simulink model "TEST"  (R2019a)
settings: Solver=VariableStepAuto  StartTime=0.0  StopTime=500  RelTol=1e-3
undefined symbols (not defined in the file): A, As, c, Cd, f, G, J, JD_0, Jw, Ks, L, Ls, M, m_max, q, r_ecef, t_orbit, v_ecef
libraries: vrlib x7, dspmathops x1, simulink_extras x1
(part 1 of 2)
settings Model: Creator=mario  LastModifiedBy=mario
settings DataIOCC: ReturnWorkspaceOutputs=off
settings DebuggingCC: ArithmeticOperatorsInVariantConditions=warning

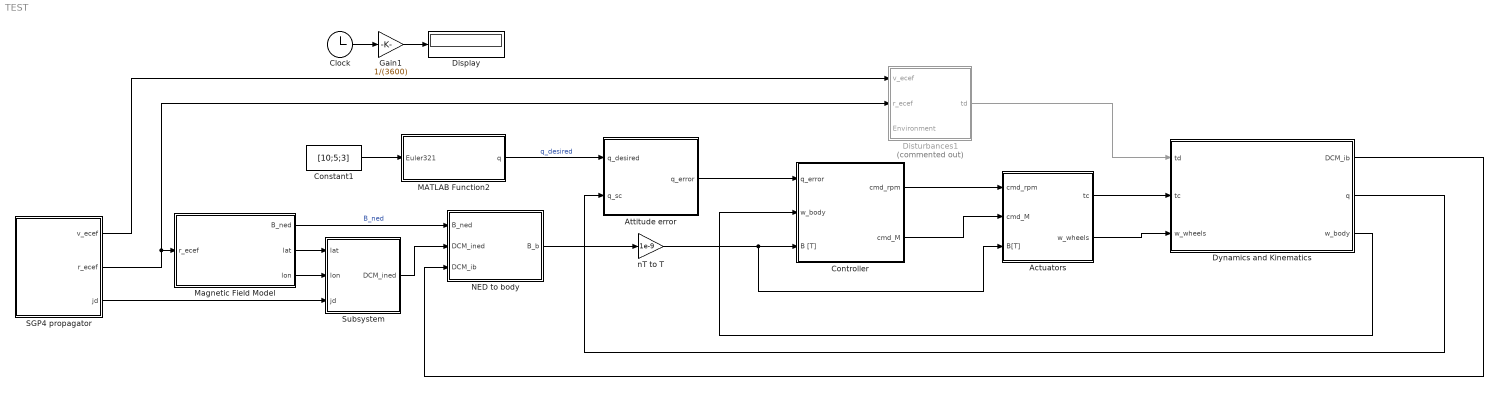
== system TEST ==
  Actuators : Subsystem
  Attitude error : Subsystem
  Clock : Clock
  Constant1 : Constant  Value=[10;5;3]
  Controller : Subsystem
  Display : Display
  Disturbances1 : Subsystem  Commented=on
  "Dynamics and Kinematics " : Subsystem
  Gain1 : Gain  Gain=1/(3600)
  MATLAB Function2 : MATLAB Function  TreatAsAtomicUnit=on
  Magnetic Field Model : Subsystem
  NED to body : Subsystem
  SGP4 propagator : Subsystem
  Subsystem : Subsystem
  nT to T : Gain  Gain=1e-9
  wires:
  "Dynamics and Kinematics "/2(q) -> Attitude error/2(q_sc)
  Constant1/1 -> MATLAB Function2/1(Euler321)
  MATLAB Function2/1(q) -> Attitude error/1(q_desired)  "q_desired"
  Controller/1("cmd_rpm ") -> Actuators/1(cmd_rpm)
  Actuators/1(tc) -> "Dynamics and Kinematics "/2(tc)
  Actuators/2(w_wheels) -> "Dynamics and Kinematics "/3(w_wheels)
  "Dynamics and Kinematics "/3(w_body) -> Controller/2(w_body)
  Attitude error/1("q_error ") -> Controller/1(q_error)
  Controller/2(cmd_M) -> Actuators/2(cmd_M)
  NED to body/1(B_b) -> nT to T/1
  nT to T/1 -> Actuators/3(B[T]), Controller/3(B [T])
  Clock/1 -> Gain1/1
  Gain1/1 -> Display/1
  Disturbances1/1(td) -> "Dynamics and Kinematics "/1(td)
  SGP4 propagator/2(r_ecef) -> Disturbances1/2("r_ecef "), Magnetic Field Model/1(r_ecef)
  "Dynamics and Kinematics "/1(DCM_ib) -> NED to body/3(DCM_ib)
  Magnetic Field Model/1(B_ned) -> NED to body/1(B_ned)  "B_ned"
  Magnetic Field Model/2(lat) -> Subsystem/1(lat)
  Magnetic Field Model/3(lon) -> Subsystem/2(lon)
  Subsystem/1(DCM_ined) -> NED to body/2(DCM_ined)
  SGP4 propagator/3(jd) -> Subsystem/3(jd)
  SGP4 propagator/1(v_ecef) -> Disturbances1/1(v_ecef)

== system TEST/Actuators ==
  cmd_rpm : Inport
  cmd_M : Inport  Port=2
  B[T] : Inport  Port=3
  Gain : Gain  Gain=0
  Magnetorquers : Subsystem
  Reaction Wheels : Subsystem
  Scope : Scope
  Sum : Sum
  tc : Outport  VectorParamsAs1DForOutWhenUnconnected=on
  w_wheels : Outport  Port=2  VectorParamsAs1DForOutWhenUnconnected=on
  wires:
  Reaction Wheels/1(t_wheels) -> Gain/1
  Reaction Wheels/2(w_wheels) -> w_wheels/1
  Magnetorquers/1(t_mtq) -> Sum/2
  Sum/1 -> Scope/1, tc/1
  cmd_rpm/1 -> Reaction Wheels/1(cmd_rpm)
  cmd_M/1 -> Magnetorquers/1(cmd_Mag)
  B[T]/1 -> Magnetorquers/2(B [T])
  Gain/1 -> Sum/1

== system TEST/Attitude error ==
  q_desired : Inport
  q_sc : Inport  Port=2
  Demux : Demux
  Gain : Gain  Gain=[1 0 0 0;0 -1 0 0;0 0 -1 0;0 0 0 -1]  Multiplication=Matrix(K*u)
  Matrix Multiply : Product  Multiplication=Matrix(*)
  Q : Subsystem
  Out Bus Element : Outport  PortName=q_error  Element=q0
  Out Bus Element1 : Outport  PortName=q_error  Element=q1
  Out Bus Element2 : Outport  PortName=q_error  Element=q2
  Out Bus Element3 : Outport  PortName=q_error  Element=q3
  wires:
  q_desired/1 -> Q/1(q)
  q_sc/1 -> Gain/1
  Q/1(Q(q)) -> Matrix Multiply/1
  Gain/1 -> Matrix Multiply/2
  Matrix Multiply/1 -> Demux/1
  Demux/1 -> Out Bus Element/1
  Demux/3 -> Out Bus Element2/1
  Demux/2 -> Out Bus Element1/1
  Demux/4 -> Out Bus Element3/1

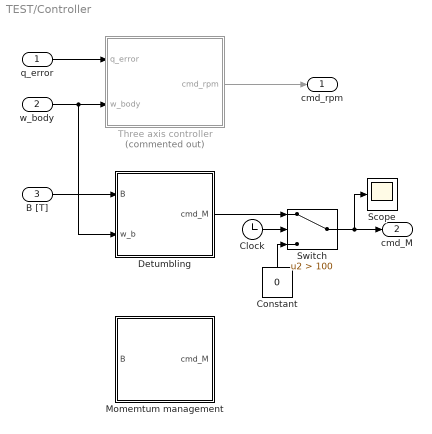
== system TEST/Controller ==
  q_error : Inport
  w_body : Inport  Port=2
  B [T] : Inport  Port=3
  Clock : Clock
  Constant : Constant  Value=0
  Detumbling : Subsystem
  Momemtum management : Subsystem
  Scope : Scope
  Switch : Switch  Criteria=u2 > Threshold  Threshold=100
  Three axis controller : Subsystem  Commented=on
  "cmd_rpm " : Outport
  cmd_M : Outport  Port=2
  wires:
  w_body/1 -> Detumbling/2(w_b), Three axis controller/2(w_body)
  q_error/1 -> Three axis controller/1(q_error)
  Three axis controller/1(cmd_rpm) -> "cmd_rpm "/1
  Detumbling/1(cmd_M) -> Switch/1
  B [T]/1 -> Detumbling/1(B)
  Switch/1 -> Scope/1, cmd_M/1
  Clock/1 -> Switch/2
  Constant/1 -> Switch/3

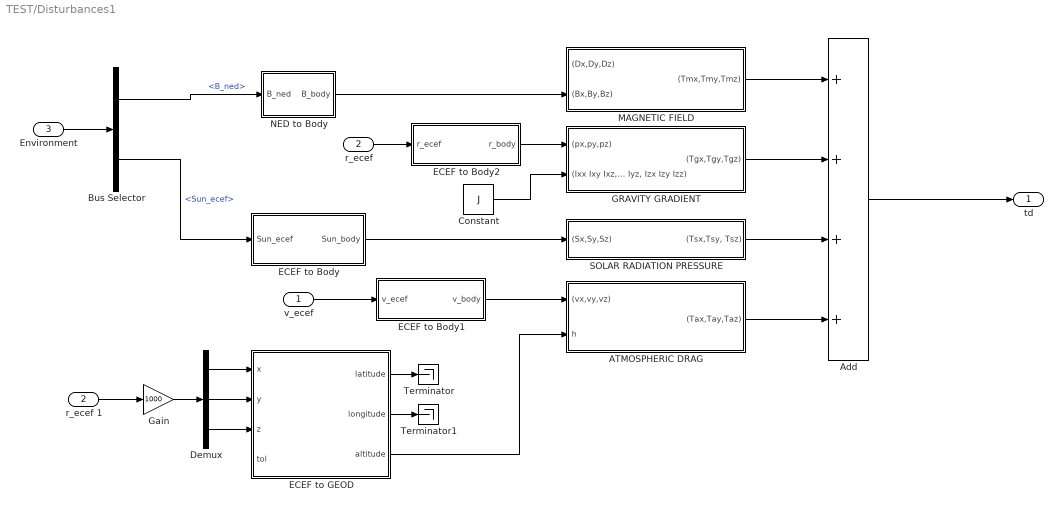
== system TEST/Disturbances1 ==
  v_ecef : Inport
  "r_ecef " : Inport  Port=2
  Environment : Inport  Port=3
  ATMOSPHERIC DRAG : Subsystem
  Add : Sum  Inputs=4
  Bus Selector : BusSelector  OutputSignals=B_ned,Sun_ecef
  Constant : Constant  Value=J
  Demux : Demux  Outputs=3
  ECEF to Body : Subsystem
  ECEF to Body1 : Subsystem
  ECEF to Body2 : Subsystem
  ECEF to GEOD : MATLAB Function  TreatAsAtomicUnit=on
  GRAVITY GRADIENT : Subsystem
  Gain : Gain  Gain=1000
  "MAGNETIC FIELD " : Subsystem
  NED to Body : Subsystem
  SOLAR RADIATION PRESSURE : Subsystem
  Terminator : Terminator
  Terminator1 : Terminator
  r_ecef 1 : InportShadow  Port=2
  td : Outport
  wires:
  Add/1 -> td/1
  ECEF to GEOD/3(altitude) -> ATMOSPHERIC DRAG/2("h ")
  Constant/1 -> GRAVITY GRADIENT/2("(Ixx Ixy Ixz, Iyx Iyy Iyz, Izx Izy Izz)")
  ATMOSPHERIC DRAG/1((Tax,Tay,Taz)) -> Add/4
  GRAVITY GRADIENT/1((Tgx,Tgy,Tgz)) -> Add/2
  ? -> "MAGNETIC FIELD "/1((Dx,Dy,Dz))
  SOLAR RADIATION PRESSURE/1("(Tsx,Tsy, Tsz)") -> Add/3
  NED to Body/1(B_body) -> "MAGNETIC FIELD "/2((Bx,By,Bz))
  "MAGNETIC FIELD "/1((Tmx,Tmy,Tmz)) -> Add/1
  ECEF to Body/1(Sun_body) -> SOLAR RADIATION PRESSURE/1((Sx,Sy,Sz))
  ECEF to Body1/1(v_body) -> ATMOSPHERIC DRAG/1((vx,vy,vz))
  Environment/1 -> Bus Selector/1
  Bus Selector/1 -> NED to Body/1(B_ned)  "<B_ned>"
  Bus Selector/2 -> ECEF to Body/1(Sun_ecef)  "<Sun_ecef>"
  v_ecef/1 -> ECEF to Body1/1(v_ecef)
  "r_ecef "/1 -> ECEF to Body2/1(r_ecef)
  ECEF to Body2/1(r_body) -> GRAVITY GRADIENT/1((px,py,pz))
  r_ecef 1/1 -> Gain/1
  Demux/1 -> ECEF to GEOD/1(x)
  Demux/2 -> ECEF to GEOD/2(y)
  Demux/3 -> ECEF to GEOD/3(z)
  ECEF to GEOD/1(latitude) -> Terminator/1
  ECEF to GEOD/2(longitude) -> Terminator1/1
  Gain/1 -> Demux/1

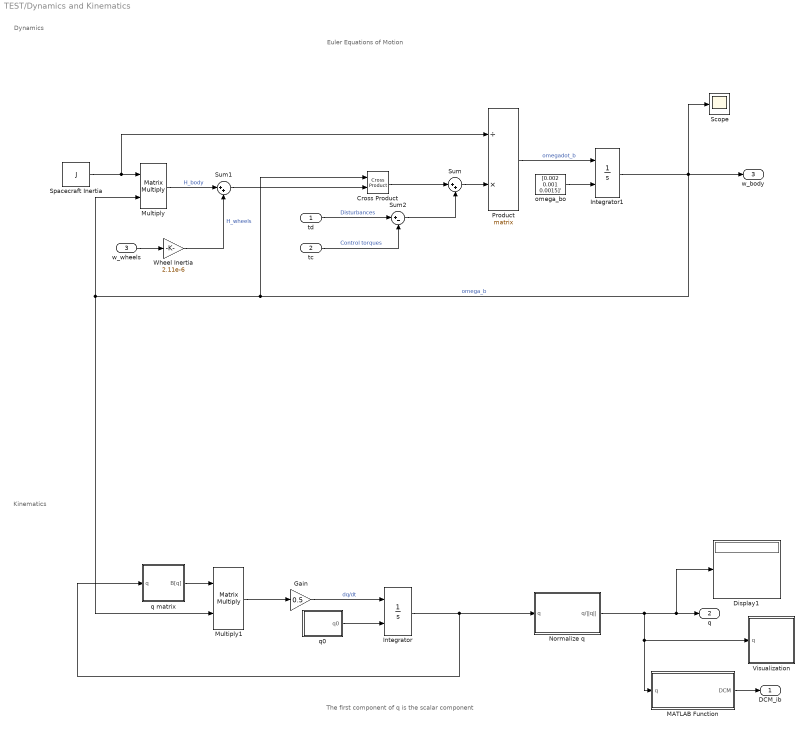
== system TEST/Dynamics and Kinematics  ==
  note: The first component of q is the scalar component
  note: Euler Equations of Motion
  note: Dynamics
  note: Kinematics
  td : Inport
  tc : Inport  Port=2
  w_wheels : Inport  Port=3
  Cross Product : vrlib/Utilities/Cross Product
      settings: SourceProductName=Simulink
  Display1 : Display
  Gain : Gain  Gain=0.5
  Integrator : Integrator  InitialConditionSource=external
  Integrator1 : Integrator  InitialConditionSource=external
  MATLAB Function : MATLAB Function  TreatAsAtomicUnit=on
  Multiply : Product  Multiplication=Matrix(*)
  Multiply1 : Product  Multiplication=Matrix(*)
  Normalize q : Subsystem
  Product : Product  Inputs=/*  Multiplication=Matrix(*)
  Scope : Scope
  Spacecraft Inertia : Constant  Value=J
  Sum : Sum  Inputs=|++
  Sum1 : Sum  Inputs=|++
  Sum2 : Sum  Inputs=|+-
  Visualization : Subsystem
  Wheel Inertia : Gain  Gain=2.11e-6
  omega_bo : Constant  Value=[0.002 0.001 0.0015]'
  q matrix : Subsystem
  q0 : Subsystem
  DCM_ib : Outport
  q : Outport  Port=2
  w_body : Outport  Port=3
  wires:
  q matrix/1(B[q]) -> Multiply1/1
  Integrator/1 -> q matrix/1(q), Normalize q/1(q)
  Gain/1 -> Integrator/1  "dq/dt"
  Multiply1/1 -> Gain/1
  Sum2/1 -> Sum/2
  Wheel Inertia/1 -> Sum1/2  "H_wheels"
  Sum1/1 -> Cross Product/2
  Cross Product/1 -> Sum/1
  Sum/1 -> Product/2
  Multiply/1 -> Sum1/1  "H_body"
  Product/1 -> Integrator1/1  "omegadot_b"
  omega_bo/1 -> Integrator1/2
  Spacecraft Inertia/1 -> Multiply/1, Product/1
  Integrator1/1 -> Scope/1, w_body/1, Multiply1/2, Multiply/2, Cross Product/1  "omega_b"
  Normalize q/1(q/||q||) -> Visualization/1(q), MATLAB Function/1(q), Display1/1, q/1
  q0/1(q0) -> Integrator/2
  td/1 -> Sum2/1  "Disturbances"
  tc/1 -> Sum2/2  "Control torques"
  w_wheels/1 -> Wheel Inertia/1
  MATLAB Function/1(DCM) -> DCM_ib/1

== system TEST/Magnetic Field Model ==
  r_ecef : Inport
  Demux : Demux  Outputs=3
  ECEF to GEOD : MATLAB Function  TreatAsAtomicUnit=on
  IGRF 13th Gen. : MATLAB Function  TreatAsAtomicUnit=on
  Mux : Mux  Inputs=3
  km to m : Gain  Gain=1000
  norm : Subsystem
  B_ned : Outport  VectorParamsAs1DForOutWhenUnconnected=on
  lat : Outport  Port=2
  lon : Outport  Port=3
  wires:
  IGRF 13th Gen./2(Be) -> Mux/2
  IGRF 13th Gen./3(Bd) -> Mux/3
  ECEF to GEOD/2(longitude) -> lon/1, IGRF 13th Gen./2(longitude)
  Demux/2 -> ECEF to GEOD/2(y)
  IGRF 13th Gen./1(Bn) -> Mux/1
  ECEF to GEOD/1(latitude) -> lat/1, IGRF 13th Gen./1(latitude)
  Demux/3 -> ECEF to GEOD/3(z)
  Demux/1 -> ECEF to GEOD/1(x)
  Mux/1 -> B_ned/1
  km to m/1 -> Demux/1
  norm/1(Out1) -> IGRF 13th Gen./3(altitude)
  r_ecef/1 -> norm/1(In1), km to m/1

== system TEST/NED to body ==
  B_ned : Inport
  DCM_ined : Inport  Port=2
  DCM_ib : Inport  Port=3
  Matrix Multiply : Product  Multiplication=Matrix(*)
  Matrix Multiply1 : Product  Multiplication=Matrix(*)
  Transpose : Math  Operator=transpose  SaturateOnIntegerOverflow=on
  B_b : Outport
  wires:
  Matrix Multiply/1 -> B_b/1
  B_ned/1 -> Matrix Multiply/2
  DCM_ib/1 -> Matrix Multiply1/1
  DCM_ined/1 -> Transpose/1
  Transpose/1 -> Matrix Multiply1/2  "DCM_nedi"
  Matrix Multiply1/1 -> Matrix Multiply/1

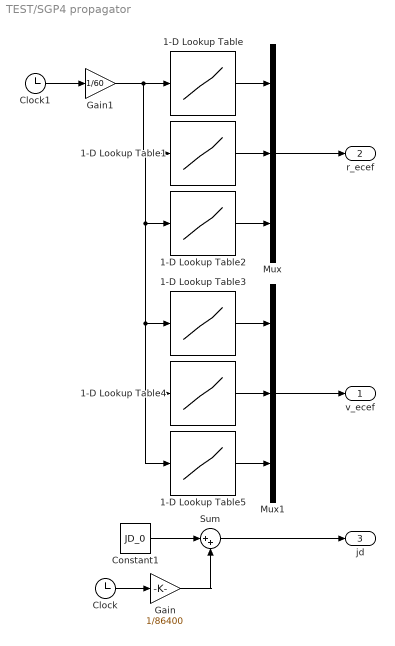
== system TEST/SGP4 propagator ==
  1-D Lookup Table : Lookup_n-D  NumberOfTableDimensions=1  BreakpointsForDimension1=t_orbit  BreakpointsForDimension2=t_orbit  BreakpointsForDimension3=t_orbit  Table=r_ecef(:,1)  InternalRulePriority=Speed  RndMeth=Simplest  InputSameDT=on
  1-D Lookup Table1 : Lookup_n-D  NumberOfTableDimensions=1  BreakpointsForDimension1=t_orbit  BreakpointsForDimension2=t_orbit  BreakpointsForDimension3=t_orbit  Table=r_ecef(:,2)  InternalRulePriority=Speed  RndMeth=Simplest  InputSameDT=on
  1-D Lookup Table2 : Lookup_n-D  NumberOfTableDimensions=1  BreakpointsForDimension1=t_orbit  BreakpointsForDimension2=t_orbit  BreakpointsForDimension3=t_orbit  Table=r_ecef(:,3)  InternalRulePriority=Speed  RndMeth=Simplest  InputSameDT=on
  1-D Lookup Table3 : Lookup_n-D  NumberOfTableDimensions=1  BreakpointsForDimension1=t_orbit  BreakpointsForDimension2=t_orbit  BreakpointsForDimension3=t_orbit  Table=v_ecef(:,1)  InternalRulePriority=Speed  RndMeth=Simplest  InputSameDT=on
  1-D Lookup Table4 : Lookup_n-D  NumberOfTableDimensions=1  BreakpointsForDimension1=t_orbit  BreakpointsForDimension2=t_orbit  BreakpointsForDimension3=t_orbit  Table=v_ecef(:,2)  InternalRulePriority=Speed  RndMeth=Simplest  InputSameDT=on
  1-D Lookup Table5 : Lookup_n-D  NumberOfTableDimensions=1  BreakpointsForDimension1=t_orbit  BreakpointsForDimension2=t_orbit  BreakpointsForDimension3=t_orbit  Table=v_ecef(:,3)  InternalRulePriority=Speed  RndMeth=Simplest  InputSameDT=on
  Clock : Clock
  Clock1 : Clock
  Constant1 : Constant  Value=JD_0
  Gain : Gain  Gain=1/86400
  Gain1 : Gain  Gain=1/60
  Mux : Mux  Inputs=3
  Mux1 : Mux  Inputs=3
  Sum : Sum  Inputs=|++
  v_ecef : Outport
  r_ecef : Outport  Port=2  VectorParamsAs1DForOutWhenUnconnected=on
  jd : Outport  Port=3
  wires:
  1-D Lookup Table2/1 -> Mux/3
  Gain1/1 -> 1-D Lookup Table5/1, 1-D Lookup Table4/1, 1-D Lookup Table3/1, 1-D Lookup Table2/1, 1-D Lookup Table1/1, 1-D Lookup Table/1
  Clock1/1 -> Gain1/1
  1-D Lookup Table1/1 -> Mux/2
  1-D Lookup Table/1 -> Mux/1
  Mux/1 -> r_ecef/1
  1-D Lookup Table3/1 -> Mux1/1
  1-D Lookup Table4/1 -> Mux1/2
  1-D Lookup Table5/1 -> Mux1/3
  Mux1/1 -> v_ecef/1
  Sum/1 -> jd/1
  Gain/1 -> Sum/2
  Constant1/1 -> Sum/1
  Clock/1 -> Gain/1

== system TEST/Subsystem ==
  lat : Inport
  lon : Inport  Port=2
  jd : Inport  Port=3
  Local Sidereal Time : MATLAB Function  TreatAsAtomicUnit=on
  MATLAB Function1 : MATLAB Function  TreatAsAtomicUnit=on
  Terminator : Terminator
  DCM_ined : Outport
  wires:
  MATLAB Function1/1(DCM_ined) -> DCM_ined/1
  Local Sidereal Time/1(lst) -> MATLAB Function1/2(lon_i)
  lat/1 -> MATLAB Function1/1(lat_d)
  lon/1 -> Local Sidereal Time/1(lon)
  jd/1 -> Local Sidereal Time/2(jd)
  Local Sidereal Time/2(gst) -> Terminator/1

== system TEST/Actuators/Magnetorquers ==
  cmd_Mag : Inport
  B [T] : Inport  Port=2
  Cross Product : vrlib/Utilities/Cross Product
      settings: SourceProductName=Simulink
  Saturation : Saturate  UpperLimit=m_max+10  LowerLimit=-m_max-10
  Scope : Scope
  Scope1 : Scope
  t_mtq : Outport
  wires:
  B [T]/1 -> Cross Product/2
  Cross Product/1 -> Scope/1, t_mtq/1
  cmd_Mag/1 -> Saturation/1
  Saturation/1 -> Scope1/1, Cross Product/1

== system TEST/Actuators/Reaction Wheels ==
  cmd_rpm : Inport
  Demux : Demux  Outputs=3
  Mux : Mux  Inputs=3
  Mux1 : Mux  Inputs=3
  Reactionwheel_x : Subsystem
  Reactionwheel_y : Subsystem
  Reactionwheel_z : Subsystem
  t_wheels : Outport
  w_wheels : Outport  Port=2
  wires:
  Reactionwheel_y/1(t_wheels) -> Mux/2
  Reactionwheel_y/2(w_wheels) -> Mux1/2
  Demux/1 -> Reactionwheel_x/1(cmd_rpm)
  Reactionwheel_x/2(w_wheels) -> Mux1/1
  Demux/2 -> Reactionwheel_y/1(cmd_rpm)
  Demux/3 -> Reactionwheel_z/1(cmd_rpm)
  Reactionwheel_z/2(w_wheels) -> Mux1/3
  Reactionwheel_x/1(t_wheels) -> Mux/1
  Reactionwheel_z/1(t_wheels) -> Mux/3
  Mux1/1 -> w_wheels/1
  Mux/1 -> t_wheels/1
  cmd_rpm/1 -> Demux/1

== system TEST/Attitude error/Q ==
  q : Inport
  Gain : Gain  Gain=[1 0 0 0;0 1 0 0;0 0 1 0;0 0 0 1]  Multiplication=Matrix(K*u)
  Gain1 : Gain  Gain=[1 0 0 0;0 -1 0 0;0 0 -1 0;0 0 0 1]  Multiplication=Matrix(K*u)
  Gain2 : Gain  Gain=[1 0 0 0;0 -1 0 0;0 0 1 0;0 0 0 -1]  Multiplication=Matrix(K*u)
  Gain4 : Gain  Gain=[1 0 0 0;0 1 0 0;0 0 -1 0;0 0 0 -1]  Multiplication=Matrix(K*u)
  Matrix Concatenate : Concatenate  NumInputs=4  Mode=Multidimensional array  ConcatenateDimension=2
  Selector1 : Selector  InputPortWidth=4  IndexOptions=Index vector (dialog)  Indices=[4 3 2 1]  OutputSizes=1
  Selector2 : Selector  InputPortWidth=4  IndexOptions=Index vector (dialog)  Indices=[2 1 4 3]  OutputSizes=1
  Selector4 : Selector  InputPortWidth=4  IndexOptions=Index vector (dialog)  Indices=[3 4 1 2]  OutputSizes=1
  Q(q) : Outport
  wires:
  Gain1/1 -> Selector2/1
  Gain/1 -> Matrix Concatenate/1
  q/1 -> Gain2/1, Gain4/1, Gain1/1, Gain/1
  Selector4/1 -> Matrix Concatenate/3
  Matrix Concatenate/1 -> Q(q)/1
  Selector2/1 -> Matrix Concatenate/2
  Gain4/1 -> Selector4/1
  Gain2/1 -> Selector1/1
  Selector1/1 -> Matrix Concatenate/4

== system TEST/Controller/Detumbling ==
  B : Inport
  w_b : Inport  Port=2
  Bang-Bang : Subsystem
  Cross Product : vrlib/Utilities/Cross Product
      settings: SourceProductName=Simulink
  Divide : Product  Inputs=*/
  Gain : Gain  Gain=-1
  Scope : Scope
  Scope1 : Scope
  norm : Subsystem
  cmd_M : Outport
  wires:
  Bang-Bang/1(Out1) -> Scope/1
  B/1 -> Cross Product/2, norm/1(B), Bang-Bang/1(In1)
  w_b/1 -> Cross Product/1
  norm/1(||B||) -> Divide/2
  Cross Product/1 -> Divide/1
  Divide/1 -> Gain/1
  Gain/1 -> cmd_M/1, Scope1/1

== system TEST/Controller/Momemtum management ==
  B : Inport
  Sign : Signum
  cmd_M : Outport

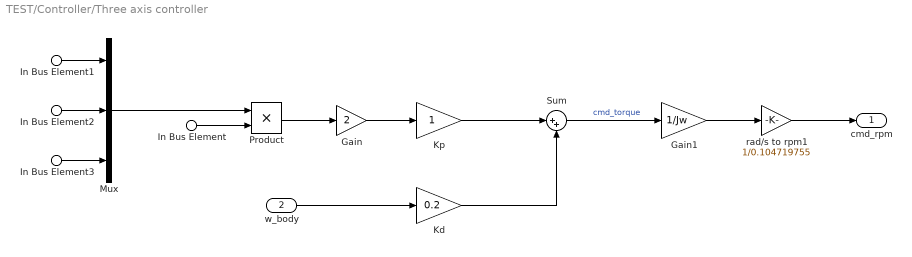
== system TEST/Controller/Three axis controller ==
  In Bus Element : Inport  PortName=q_error  Element=q0
  In Bus Element1 : Inport  PortName=q_error  Element=q1
  In Bus Element2 : Inport  PortName=q_error  Element=q2
  In Bus Element3 : Inport  PortName=q_error  Element=q3
  w_body : Inport  Port=2
  Gain : Gain  Gain=2
  Gain1 : Gain  Gain=1/Jw
  Kd : Gain  Gain=0.2
  Kp : Gain
  Mux : Mux  Inputs=3
  Product : Product
  Sum : Sum  Inputs=|++
  rad/s to rpm1 : Gain  Gain=1/0.104719755
  cmd_rpm : Outport
  wires:
  Kp/1 -> Sum/1
  w_body/1 -> Kd/1
  Product/1 -> Gain/1
  Sum/1 -> Gain1/1  "cmd_torque"
  Kd/1 -> Sum/2
  Gain1/1 -> rad/s to rpm1/1
  rad/s to rpm1/1 -> cmd_rpm/1
  Gain/1 -> Kp/1
  Mux/1 -> Product/1
  In Bus Element3/1 -> Mux/3
  In Bus Element/1 -> Product/2
  In Bus Element1/1 -> Mux/1
  In Bus Element2/1 -> Mux/2

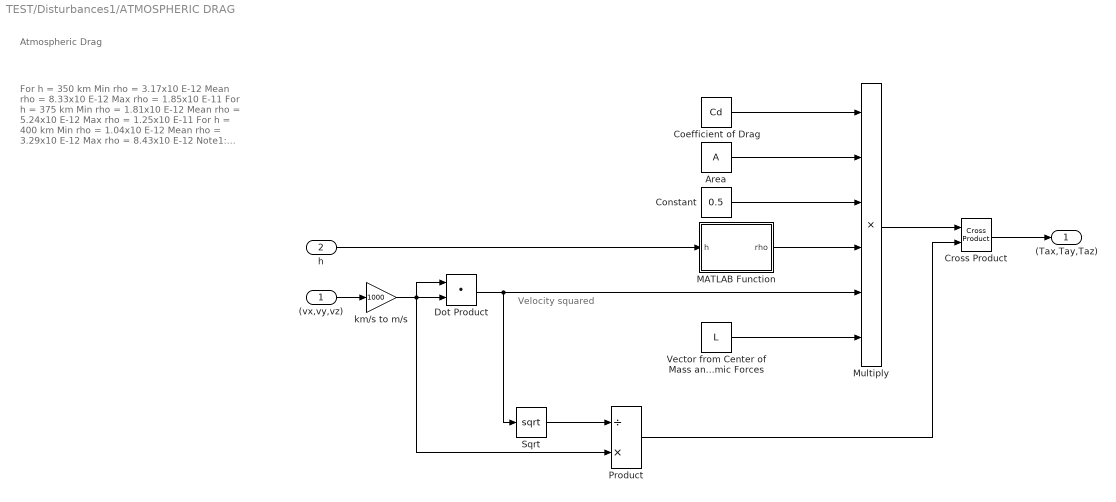
== system TEST/Disturbances1/ATMOSPHERIC DRAG ==
  note: Velocity squared
  note: For h = 350 km
      |
      | Min rho = 3.17x10 E-12
      | Mean rho = 8.33x10 E-12
      | Max rho = 1.85x10 E-11
      |
      | For h = 375 km
      |
      | Min rho = 1.81x10 E-12
      | Mean rho = 5.24x10 E-12
      | Max rho = 1.25x10 E-11
      |
      | For h = 400 km
      |
      | Min rho = 1.04x10 E-12
      | Mean rho = 3.29x10 E-12
      | Max rho = 8.43x10 E-12
      |
      | Note1: Mean Rho has an accuracy of 10%
      | Note2: Rho (kg/m^3)
      | Note3 : Rho depends on solar pressure and the solar cycle
      | Source : New SMAD p.1031
  note: Atmospheric Drag
  (vx,vy,vz) : Inport
  "h " : Inport  Port=2
  Area : Constant  Value=A
  Coefficient of Drag : Constant  Value=Cd
  Constant : Constant  Value=0.5
  Cross Product : vrlib/Utilities/Cross Product
      settings: SourceProductBaseCode=VR
  Dot Product : DotProduct  InputSameDT=on  OutDataTypeStr=Inherit: Inherit via internal rule
  MATLAB Function : MATLAB Function  TreatAsAtomicUnit=on
  Multiply : Product  Inputs=6
  Product : Product  Inputs=/*
  Sqrt : Sqrt  SaturateOnIntegerOverflow=on
  "Vector from Center of Mass and Center of Aerodynamic Forces " : Constant  Value=L
  km/s to m/s : Gain  Gain=1000
  (Tax,Tay,Taz) : Outport
  wires:
  Constant/1 -> Multiply/3
  Multiply/1 -> Cross Product/1
  (vx,vy,vz)/1 -> km/s to m/s/1
  "h "/1 -> MATLAB Function/1(h)
  Sqrt/1 -> Product/1
  Product/1 -> Cross Product/2
  Dot Product/1 -> Sqrt/1, Multiply/5
  Area/1 -> Multiply/2
  Coefficient of Drag/1 -> Multiply/1
  MATLAB Function/1(rho) -> Multiply/4
  "Vector from Center of Mass and Center of Aerodynamic Forces "/1 -> Multiply/6
  Cross Product/1 -> (Tax,Tay,Taz)/1
  km/s to m/s/1 -> Dot Product/1, Product/2, Dot Product/2

== system TEST/Disturbances1/ECEF to Body ==
  Sun_ecef : Inport
  Sun_body : Outport
  wires:
  Sun_ecef/1 -> Sun_body/1

== system TEST/Disturbances1/ECEF to Body1 ==
  v_ecef : Inport
  v_body : Outport
  wires:
  v_ecef/1 -> v_body/1

== system TEST/Disturbances1/ECEF to Body2 ==
  r_ecef : Inport
  r_body : Outport
  wires:
  r_ecef/1 -> r_body/1

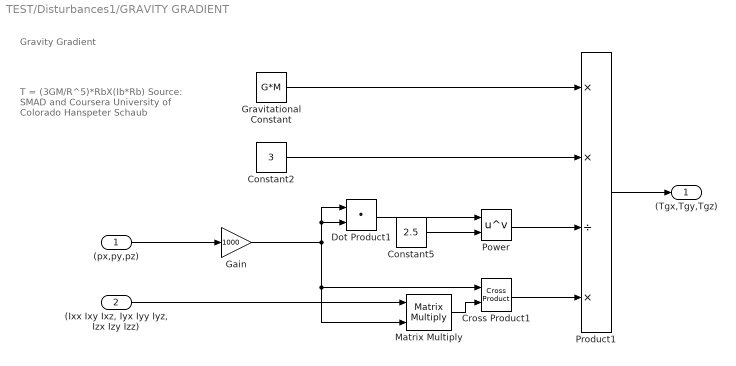
== system TEST/Disturbances1/GRAVITY GRADIENT ==
  note: T = (3GM/R^5)*RbX(Ib*Rb)
      |
      | Source: SMAD and Coursera
      | University of Colorado Hanspeter
      | Schaub
  note: Gravity Gradient
  (px,py,pz) : Inport
  "(Ixx Ixy Ixz, Iyx Iyy Iyz, Izx Izy Izz)" : Inport  Port=2
  Constant2 : Constant  Value=3
  Constant5 : Constant  Value=2.5
  Cross Product1 : vrlib/Utilities/Cross Product
      settings: SourceProductBaseCode=VR
  Dot Product1 : DotProduct  InputSameDT=on  OutDataTypeStr=Inherit: Inherit via internal rule
  Gain : Gain  Gain=1000
  Gravitational Constant : Constant  Value=G*M
  Matrix Multiply : Product  Multiplication=Matrix(*)
  Power : Math  Operator=pow  SaturateOnIntegerOverflow=on
  Product1 : Product  Inputs=**/*
  (Tgx,Tgy,Tgz) : Outport
  wires:
  (px,py,pz)/1 -> Gain/1
  Dot Product1/1 -> Power/1
  Constant5/1 -> Power/2
  Cross Product1/1 -> Product1/4
  Constant2/1 -> Product1/2
  "(Ixx Ixy Ixz, Iyx Iyy Iyz, Izx Izy Izz)"/1 -> Matrix Multiply/1
  Matrix Multiply/1 -> Cross Product1/2
  Gravitational Constant/1 -> Product1/1
  Power/1 -> Product1/3
  Product1/1 -> (Tgx,Tgy,Tgz)/1
  Gain/1 -> Matrix Multiply/2, Cross Product1/1, Dot Product1/1, Dot Product1/2

== system TEST/Disturbances1/MAGNETIC FIELD  ==
  note: Magnetic Field
  (Dx,Dy,Dz) : Inport
  (Bx,By,Bz) : Inport  Port=2
  Cross Product : vrlib/Utilities/Cross Product
      settings: SourceProductBaseCode=VR
  nT to T : Gain  Gain=1e-9
  (Tmx,Tmy,Tmz) : Outport
  wires:
  Cross Product/1 -> (Tmx,Tmy,Tmz)/1
  (Bx,By,Bz)/1 -> nT to T/1
  (Dx,Dy,Dz)/1 -> Cross Product/1
  nT to T/1 -> Cross Product/2

== system TEST/Disturbances1/NED to Body ==
  B_ned : Inport
  B_body : Outport
  wires:
  B_ned/1 -> B_body/1

== system TEST/Disturbances1/SOLAR RADIATION PRESSURE ==
  note: Solar Radiation
      | Pressure
  (Sx,Sy,Sz) : Inport
  Cross Product2 : vrlib/Utilities/Cross Product
      settings: SourceProductBaseCode=VR
  Inverse because the Force is in the opposite direction : Gain  Gain=-1
  Normalization : dspmathops/Normalization  NormType=2-norm  Bias=1e-10  NormOver=Each column  Dimension=1  roundingMode=Floor  overflowMode=off  accumDataTypeStr=Inherit: Same as product output  accumLastDataTypeStr=Inherit: Same as product output  outputDataTypeStr=Inherit: Same as product output  outputMin=[]  outputMax=[]  outputLastDataTypeStr=Inherit: Same as product output
      settings: SourceProductName=DSP System Toolbox
  Product3 : Product  Inputs=5
  Solar Constant : Constant  Value=Ks
  Speed of Light : Constant  Value=1/c
  Sunlit Area : Constant  Value=As
  Unitless Reflectance Factor : Constant  Value=1+q
  Vector from Center of Mass to Center of Solar Pressure : Constant  Value=Ls
  "(Tsx,Tsy, Tsz)" : Outport
  wires:
  Cross Product2/1 -> "(Tsx,Tsy, Tsz)"/1
  Sunlit Area/1 -> Product3/1
  Vector from Center of Mass to Center of Solar Pressure/1 -> Cross Product2/1
  (Sx,Sy,Sz)/1 -> Normalization/1
  Solar Constant/1 -> Product3/4
  Product3/1 -> Cross Product2/2
  Inverse because the Force is in the opposite direction/1 -> Product3/5
  Speed of Light/1 -> Product3/3
  Unitless Reflectance Factor/1 -> Product3/2
  Normalization/1 -> Inverse because the Force is in the opposite direction/1

== system TEST/Dynamics and Kinematics /Normalize q ==
  q : Inport
  Divide : Product  Inputs=*/
  Dot Product : DotProduct  InputSameDT=on  OutDataTypeStr=Inherit: Inherit via internal rule
  Sqrt : Sqrt  SaturateOnIntegerOverflow=on
  q/||q|| : Outport
  wires:
  Divide/1 -> q/||q||/1
  Dot Product/1 -> Sqrt/1
  Sqrt/1 -> Divide/2
  q/1 -> Dot Product/1, Dot Product/2, Divide/1

== system TEST/Dynamics and Kinematics /Visualization ==
  q : Inport
  MATLAB Function : MATLAB Function  TreatAsAtomicUnit=on
  Radians to Degrees : simulink_extras/Transformations/Radians to Degrees
  Scope : Scope
  To Workspace : ToWorkspace  VariableName=euler  SampleTime=0.05
  wires:
  Radians to Degrees/1 -> Scope/1
  MATLAB Function/1(Euler321) -> Radians to Degrees/1, To Workspace/1
  q/1 -> MATLAB Function/1(q)

== system TEST/Dynamics and Kinematics /q matrix ==
  q : Inport
  Gain : Gain  Gain=[1 0 0 0;0 -1 0 0;0 0 -1 0;0 0 0 1]  Multiplication=Matrix(K*u)
  Gain1 : Gain  Gain=[1 0 0 0;0 1 0 0;0 0 -1 0;0 0 0 -1]  Multiplication=Matrix(K*u)
  Gain4 : Gain  Gain=[1 0 0 0;0 -1 0 0;0 0 1 0;0 0 0 -1]  Multiplication=Matrix(K*u)
  Matrix Concatenate : Concatenate  NumInputs=3  Mode=Multidimensional array  ConcatenateDimension=2
  Selector : Selector  InputPortWidth=4  IndexOptions=Index vector (dialog)  Indices=[2 1 4 3]  OutputSizes=1
  Selector2 : Selector  InputPortWidth=4  IndexOptions=Index vector (dialog)  Indices=[3 4 1 2]  OutputSizes=1
  Selector4 : Selector  InputPortWidth=4  IndexOptions=Index vector (dialog)  Indices=[4 3 2 1]  OutputSizes=1
  B[q] : Outport
  wires:
  Gain/1 -> Selector/1
  Gain1/1 -> Selector2/1
  Selector/1 -> Matrix Concatenate/1
  q/1 -> Gain1/1, Gain/1, Gain4/1
  Selector4/1 -> Matrix Concatenate/3
  Matrix Concatenate/1 -> B[q]/1
  Selector2/1 -> Matrix Concatenate/2
  Gain4/1 -> Selector4/1

== system TEST/Dynamics and Kinematics /q0 ==
  Constant : Constant  Value=[0;0;0]
  MATLAB Function1 : MATLAB Function  TreatAsAtomicUnit=on
  q0 : Outport
  wires:
  Constant/1 -> MATLAB Function1/1(Euler321)
  MATLAB Function1/1(q) -> q0/1

== system TEST/Magnetic Field Model/norm ==
  In1 : Inport
  Add : Sum  Inputs=+++
  Demux : Demux  Outputs=3
  Product : Product
  Product1 : Product
  Product2 : Product
  Sqrt : Sqrt  SaturateOnIntegerOverflow=on
  Out1 : Outport
  wires:
  Demux/2 -> Product1/2, Product1/1
  Demux/1 -> Product/2, Product/1
  Sqrt/1 -> Out1/1
  Product2/1 -> Add/3
  Product1/1 -> Add/2
  Product/1 -> Add/1
  Add/1 -> Sqrt/1
  Demux/3 -> Product2/2, Product2/1
  In1/1 -> Demux/1

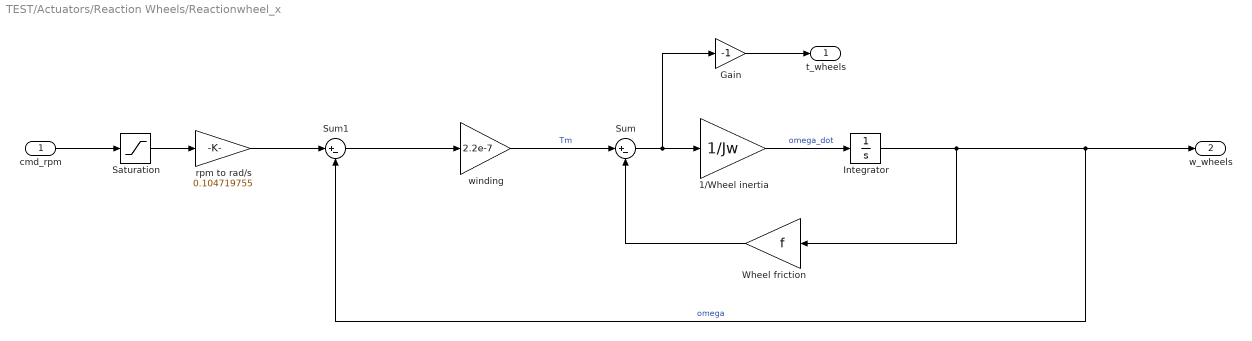
== system TEST/Actuators/Reaction Wheels/Reactionwheel_x ==
  cmd_rpm : Inport
  1/Wheel inertia : Gain  Gain=1/Jw
  Gain : Gain  Gain=-1
  Integrator : Integrator
  Saturation : Saturate  UpperLimit=8000  LowerLimit=-8000
  Sum : Sum  Inputs=|+-
  Sum1 : Sum  Inputs=|+-
  Wheel friction : Gain  Gain=f
  rpm to rad/s : Gain  Gain=0.104719755
  winding : Gain  Gain=2.2e-7
  t_wheels : Outport
  w_wheels : Outport  Port=2
  wires:
  cmd_rpm/1 -> Saturation/1
  Integrator/1 -> w_wheels/1, Sum1/2, Wheel friction/1  "omega"
  Wheel friction/1 -> Sum/2
  Sum1/1 -> winding/1
  1/Wheel inertia/1 -> Integrator/1  "omega_dot"
  winding/1 -> Sum/1  "Tm"
  Sum/1 -> Gain/1, 1/Wheel inertia/1
  rpm to rad/s/1 -> Sum1/1
  Saturation/1 -> rpm to rad/s/1
  Gain/1 -> t_wheels/1

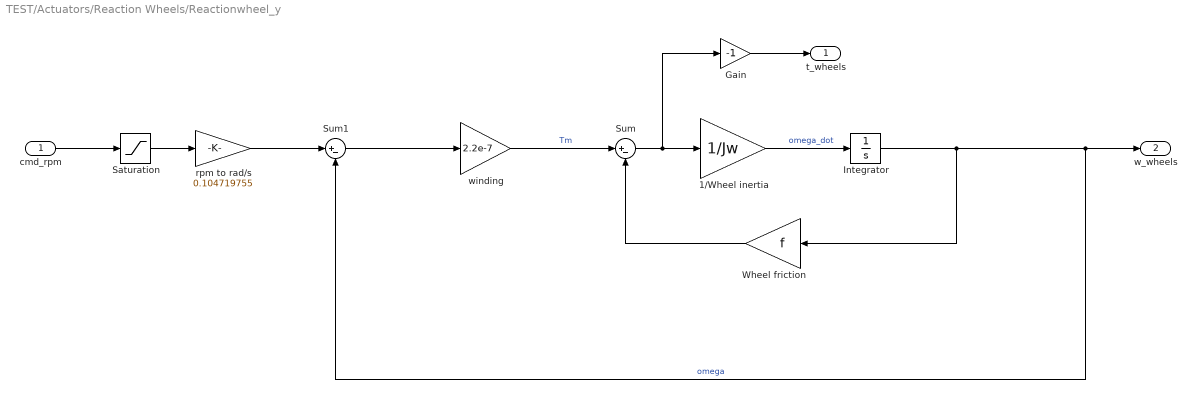
== system TEST/Actuators/Reaction Wheels/Reactionwheel_y ==
  cmd_rpm : Inport
  1/Wheel inertia : Gain  Gain=1/Jw
  Gain : Gain  Gain=-1
  Integrator : Integrator
  Saturation : Saturate  UpperLimit=8000  LowerLimit=-8000
  Sum : Sum  Inputs=|+-
  Sum1 : Sum  Inputs=|+-
  Wheel friction : Gain  Gain=f
  rpm to rad/s : Gain  Gain=0.104719755
  winding : Gain  Gain=2.2e-7
  t_wheels : Outport
  w_wheels : Outport  Port=2
  wires:
  Saturation/1 -> rpm to rad/s/1
  rpm to rad/s/1 -> Sum1/1
  Sum/1 -> 1/Wheel inertia/1, Gain/1
  winding/1 -> Sum/1  "Tm"
  1/Wheel inertia/1 -> Integrator/1  "omega_dot"
  Sum1/1 -> winding/1
  Wheel friction/1 -> Sum/2
  Integrator/1 -> Wheel friction/1, w_wheels/1, Sum1/2  "omega"
  cmd_rpm/1 -> Saturation/1
  Gain/1 -> t_wheels/1

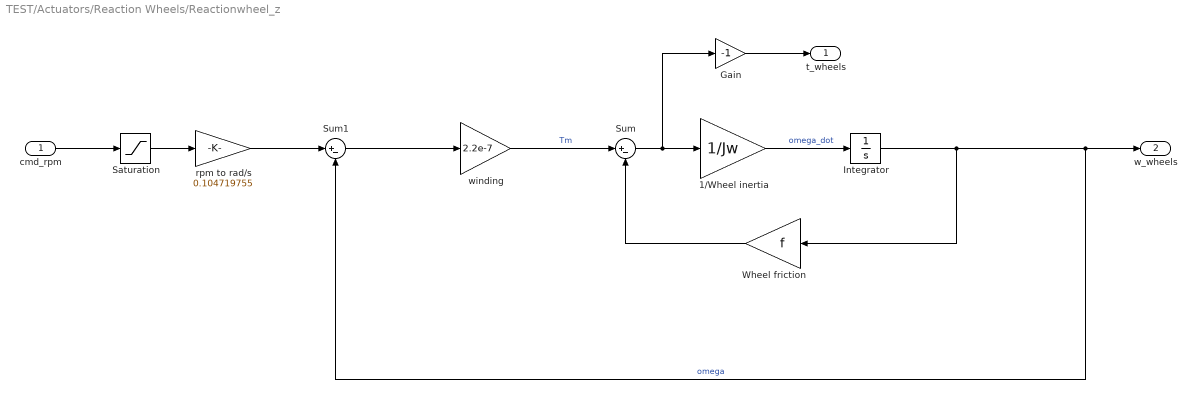
== system TEST/Actuators/Reaction Wheels/Reactionwheel_z ==
  cmd_rpm : Inport
  1/Wheel inertia : Gain  Gain=1/Jw
  Gain : Gain  Gain=-1
  Integrator : Integrator
  Saturation : Saturate  UpperLimit=8000  LowerLimit=-8000
  Sum : Sum  Inputs=|+-
  Sum1 : Sum  Inputs=|+-
  Wheel friction : Gain  Gain=f
  rpm to rad/s : Gain  Gain=0.104719755
  winding : Gain  Gain=2.2e-7
  t_wheels : Outport
  w_wheels : Outport  Port=2
  wires:
  cmd_rpm/1 -> Saturation/1
  Integrator/1 -> Sum1/2, w_wheels/1, Wheel friction/1  "omega"
  Wheel friction/1 -> Sum/2
  Sum1/1 -> winding/1
  1/Wheel inertia/1 -> Integrator/1  "omega_dot"
  winding/1 -> Sum/1  "Tm"
  Sum/1 -> Gain/1, 1/Wheel inertia/1
  rpm to rad/s/1 -> Sum1/1
  Saturation/1 -> rpm to rad/s/1
  Gain/1 -> t_wheels/1

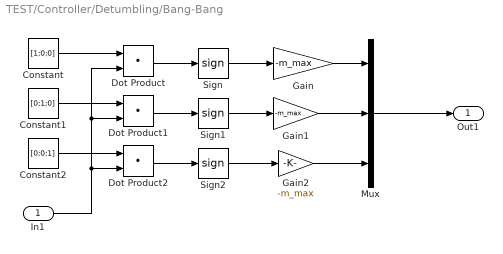
== system TEST/Controller/Detumbling/Bang-Bang ==
  In1 : Inport
  Constant : Constant  Value=[1;0;0]
  Constant1 : Constant  Value=[0;1;0]
  Constant2 : Constant  Value=[0;0;1]
  Dot Product : DotProduct  InputSameDT=on  OutDataTypeStr=Inherit: Inherit via internal rule
  Dot Product1 : DotProduct  InputSameDT=on  OutDataTypeStr=Inherit: Inherit via internal rule
  Dot Product2 : DotProduct  InputSameDT=on  OutDataTypeStr=Inherit: Inherit via internal rule
  Gain : Gain  Gain=-m_max
  Gain1 : Gain  Gain=-m_max
  Gain2 : Gain  Gain=-m_max
  Mux : Mux  Inputs=3
  Sign : Signum
  Sign1 : Signum
  Sign2 : Signum
  Out1 : Outport
  wires:
  In1/1 -> Dot Product2/2, Dot Product1/2, Dot Product/2
  Dot Product2/1 -> Sign2/1
  Sign2/1 -> Gain2/1
  Gain/1 -> Mux/1
  Sign/1 -> Gain/1
  Sign1/1 -> Gain1/1
  Constant/1 -> Dot Product/1
  Constant1/1 -> Dot Product1/1
  Dot Product/1 -> Sign/1
  Gain2/1 -> Mux/3
  Constant2/1 -> Dot Product2/1
  Dot Product1/1 -> Sign1/1
  Gain1/1 -> Mux/2
  Mux/1 -> Out1/1

== system TEST/Controller/Detumbling/norm ==
  B : Inport
  Add : Sum  Inputs=3
  Demux : Demux  Outputs=3
  Product : Product
  Product1 : Product
  Product2 : Product
  ||B|| : Outport
  wires:
  Add/1 -> ||B||/1
  Product2/1 -> Add/3
  Product1/1 -> Add/2
  Product/1 -> Add/1
  Demux/3 -> Product2/1, Product2/2
  Demux/2 -> Product1/1, Product1/2
  Demux/1 -> Product/1, Product/2
  B/1 -> Demux/1

== matlab function TEST/Dynamics and Kinematics /q0/MATLAB Function1 ==
  data: Euler321 input; q output
function q = euler3212q(Euler321)
euler = [deg2rad(Euler321(1));deg2rad(Euler321(2));deg2rad(Euler321(3))];

c1 = cos(euler(1)/2);
s1 = sin(euler(1)/2);
c2 = cos(euler(2)/2);
s2 = sin(euler(2)/2);
c3 = cos(euler(3)/2);
s3 = sin(euler(3)/2);

q = [c1*c2*c3+s1*s2*s3 ;
     s1*c2*c3-c1*s2*s3;
     c1*s2*c3+s1*c2*s3;
     c1*c2*s3-s1*s2*c3];

== matlab function TEST/Dynamics and Kinematics /Visualization/MATLAB Function ==
  data: q input; Euler321 output
function Euler321 = q2euler(q)
q1 = q(1);
qbar = [q(2);q(3);q(4)];
qtilde = [0 -qbar(3) qbar(2);qbar(3) 0 -qbar(1);-qbar(2) qbar(1) 0];

DCM = 2*(qbar*qbar') + (q1^2-qbar'*qbar)*eye(3) - 2*q1*qtilde;

Euler321 = [atan2(DCM(1,2),DCM(1,1));-asin(DCM(1,3)); atan2(DCM(2,3),DCM(3,3))];

== matlab function TEST/MATLAB Function2 ==
  data: Euler321 input; q output
function q = euler3212q(Euler321)
euler = [deg2rad(Euler321(1));deg2rad(Euler321(2));deg2rad(Euler321(3))];

c1 = cos(euler(1)/2);
s1 = sin(euler(1)/2);
c2 = cos(euler(2)/2);
s2 = sin(euler(2)/2);
c3 = cos(euler(3)/2);
s3 = sin(euler(3)/2);

q = [c1*c2*c3+s1*s2*s3 ;
     s1*c2*c3-c1*s2*s3;
     c1*s2*c3+s1*c2*s3;
     c1*c2*s3-s1*s2*c3];

== matlab function TEST/Subsystem/Local Sidereal Time ==
  data: lon input; lst output; jd input; gst output
% -----------------------------------------------------------------------------
%
%                           function lstime
%
%  this function finds the local sidereal time at a given location.
%
%  author        : david vallado                  719-573-2600   27 may 2002
%
%  revisions
%                -
%
%  inputs          description                    range / units
%    lon         - site longitude (west -)        -2pi to 2pi rad
%    jd          - julian date                    days from 4713 bc
%
%  outputs       :
%    lst         - local sidereal time            0.0 to 2pi rad
%    gst         - greenwich sidereal time        0.0 to 2pi rad
%
%  locals        :
%    none.
%
%  coupling      :
%    gstime        finds the greenwich sidereal time
%
%  references    :
%    vallado       2007, 194, alg 15, ex 3-5
%
% [lst,gst] = lstime ( lon, jd );
% -----------------------------------------------------------------------------

function [lst,gst] = lstime ( lon, jd )

        twopi  = 2.0*pi;

        % ------------------------  implementation   ------------------
        [gst] = gstime( jd );
        lst = lon + gst;

        % ----------------------- check quadrants ---------------------
        lst = rem( lst,twopi );
        if ( lst < 0.0 )
            lst= lst + twopi;
        end
          
% -----------------------------------------------------------------------------
%
%                           function gstime
%
%  this function finds the greenwich sidereal time (iau-82).
%
%  author        : david vallado                  719-573-2600    7 jun 2002
%
%  revisions
%                -
%
%  inputs          description                    range / units
%    jdut1       - julian date of ut1             days from 4713 bc
%
%  outputs       :
%    gst         - greenwich sidereal time        0 to 2pi rad
%
%  locals        :
%    temp        - temporary variable for reals   rad
%    tut1        - julian centuries from the
%                  jan 1, 2000 12 h epoch (ut1)
%
%  coupling      :
%
%  references    :
%    vallado       2007, 193, Eq 3-43
%
% gst = gstime(jdut1);
% -----------------------------------------------------------------------------

function gst = gstime(jdut1);

        twopi      = 2.0*pi;
        deg2rad    = pi/180.0;

        % ------------------------  implementation   ------------------
        tut1= ( jdut1 - 2451545.0 ) / 36525.0;

        temp = - 6.2e-6 * tut1 * tut1 * tut1 + 0.093104 * tut1 * tut1  ...
               + (876600.0 * 3600.0 + 8640184.812866) * tut1 + 67310.54841;

        % 360/86400 = 1/240, to deg, to rad
        temp = rem( temp*deg2rad/240.0,twopi );

        % ------------------------ check quadrants --------------------
        if ( temp < 0.0 )
            temp = temp + twopi;
        end

        gst = temp;

== matlab function TEST/Dynamics and Kinematics /MATLAB Function ==
  data: q input; DCM output
function DCM = q2dcm(q)
q1 = q(1);
qbar = [q(2);q(3);q(4)];
qtilde = [0 -qbar(3) qbar(2);qbar(3) 0 -qbar(1);-qbar(2) qbar(1) 0];

DCM = 2*(qbar*qbar') + (q1^2-qbar'*qbar)*eye(3) - 2*q1*qtilde;

== matlab function TEST/Magnetic Field Model/ECEF to GEOD ==
  data: x input; latitude output; y input; z input; tol input; longitude output; altitude output
function [latitude, longitude, altitude] = ecef2geod(x, y, z, tol)

% ECEF2GEOD Convert ECEF coordinates to geodetic coordinates.
% 
% Usage: [LATITUDE, LONGITUDE, ALTITUDE] = ECEF2GEOD(X, Y, Z, TOL)
%     or [LATITUDE, LONGITUDE, ALTITUDE] = ECEF2GEOD(XYZ, TOL)
%     or LLA = ECEF2GEOD(X, Y, Z, TOL)
%     or LLA = ECEF2GEOD(XYZ, TOL)
% 
% Converts Earth-centered, Earth fixed (ECEF) coordinates X, Y, and Z to
% geodetic coordinates LATITUDE, LONGITUDE, and ALTITUDE. For a matrix
% input, the first dimension with length 3 is assumed to have the three
% separate X, Y, and Z inputs across it. The World Geodetic System 1984
% (WGS84) ellipsoid model of the Earth is assumed.
% 
% Inputs:
%   -X: x coordinates of the point in meters.
%   -Y: y coordinates of the point in meters.
%   -Z: z coordinates of the point in meters.
%   -TOL: Maximum error tolerance in the latitude in radians (optional,
%   default is 1e-12).
%   -XYZ: Matrix with at least one dimension with length 3, the first of
%   which corresponding to the dimension across which the three inputs
%   above go.
% 
% Ouputs:
%   -LATITUDE: Geodetic latitude in degrees.
%   -LONGITUDE: Geodetic longitude in degrees.
%   -ALTITUDE: Height above the Earth in meters.
%   -LLA: When just one output is requested, the three outputs above are
%   returned as a row vector for scalar inputs, an M-by-3 matrix for column
%   vector inputs, a 3-by-M matrix for row vector inputs, or the three
%   outputs concatenated either along the next largest dimension when the
%   inputs are separate arguments or the same dimension that the inputs
%   went across when a single matrix is input.
% 
% See also: ECEF2LLA, GEOD2ECEF.

% Input checking.
if nargin <= 2
    error(nargchk(1, 2, nargin));
    if nargin == 1
        tol = [];
    else
        tol = y;
    end
    sizex = size(x); first3 = find(sizex == 3, 1, 'first');
    x = reshape(permute(x, [first3, 1:(first3 - 1), ...
        (first3 + 1):ndims(x)]), 3, []);
    sizex(first3) = 1;
    y = reshape(x(2, :), sizex);
    z = reshape(x(3, :), sizex);
    x = reshape(x(1, :), sizex);
else
    error(nargchk(3, 4, nargin));
end
if nargin <= 3 || isempty(tol)
    tol = 1e-12;
end

% WGS84 parameters.
a = 6378137; f = 1/298.257223563; b = a*(1 - f); e2 = 1 - (b/a)^2;

% Longitude is easy:
longitude = atan2(y, x)*180/pi;

% Compute latitude recursively.
rd = hypot(x, y);
[latitude, Nphi] = recur(asin(z ./ hypot(x, hypot(y, z))), z, a, e2, ...
    rd, tol, 1);
sinlat = sin(latitude); coslat = cos(latitude); latitude = latitude*180/pi;

% Get altitude from latitude.
altitude = rd.*coslat + (z + e2*Nphi.*sinlat).*sinlat - Nphi;

% Shape output according to number of arguments.
if nargout <= 1
    if nargin <= 2
        latitude = cat(first3, latitude, longitude, altitude);
    else
        dims = ndims(latitude);
        if dims == 2
            if size(latitude, 2) == 1
                latitude = [latitude, longitude, altitude];
            else
                latitude = [latitude; longitude; latitude];
            end
        else
            latitude = cat(dims + 1, latitude, longitude, altitude);
        end
    end
end

function [latitude, Nphi] = recur(lat_in, z, a, e2, rd, tol, iter)
thisNphi = a ./ sqrt(1 - e2*sin(lat_in).^2);
nextlat = atan((z + thisNphi*e2.*sin(lat_in))./rd);
if all(abs(lat_in - nextlat) < tol) || iter > 100
    latitude = nextlat; Nphi = thisNphi;
else
    [latitude, Nphi] = recur(nextlat, z, a, e2, rd, tol, iter + 1);
end

== matlab function TEST/Magnetic Field Model/IGRF 13th Gen. ==
  data: latitude input; Bn output; longitude input; altitude input; Be output; Bd output
function [Bn, Be, Bd] = igrf(latitude, longitude, altitude)

%REMOVED COORD AS EVERYTHING IS ALREADY IN GEOCENTRIC. KEEPING TIME FOR NOW

% IGRF Earth's magnetic field from IGRF model.
% 
% Usage: [BX, BY, BZ] = IGRF(TIME, LATITUDE, LONGITUDE, ALTITUDE, COORD)
%     or [BX, BY, BZ] = IGRF(COEFS, LATITUDE, LONGITUDE, ALTITUDE, COORD)
%     or B = IGRF(TIME, LATITUDE, LONGITUDE, ALTITUDE, COORD)
%     or B = IGRF(COEFS, LATITUDE, LONGITUDE, ALTITUDE, COORD)
% 
% Calculates the components of the Earth's magnetic field using the
% International Geomagnetic Reference Field (IGRF) model. The inputs for
% the position can be scalars or vectors (in the latter case each should
% have the same number of elements or be a scalar), but TIME must be a
% scalar.
% 
% When all the coordinate inputs are scalars, the function can be run more
% efficiently by providing the proper IGRF coefficient vector for a given
% time rather than the time itself. This mode is useful when making
% multiple calls to the function while keeping the time the same (meaning
% the coefficients will be the same for each run) as loading the
% coefficients can be the most time-consuming part of the function. The
% coefficient vector can be easily loaded using the function LOADIGRFCOEFS.
% This mode is assumed when all the coordinate inputs are scalars and the
% first input is a vector. In this case, the coefficient vector should be
% formatted as (LOADIGRFCOEFS provides this):
% 
%   [g(n=1,m=0) g(n=1,m=1) h(n=1,m=1) g(n=2,m=0) g(n=2,m=1) h(n=2,m=1) ...]
% 
% Regardless of the size of the inputs, the outputs will be column vectors.
% If only one output is requested, B = [BX(:), BY(:), BZ(:)] is output.
% Note that the other parameters the IGRF gives can be computed from BX,
% BY, and BZ as:
% 
%   Horizonal intensity: hypot(BX, BY) (i.e., sqrt(BX.^2 + BY.^2) )
%   Total intensity: hypot(BX, hypot(BY, BZ))
%   Declination: atan2(BY, BX)
%   Inclination: atan(BZ./hypot(BX, BY))
% 
% This function relies on having the file igrfcoefs.mat in the MATLAB
% path to function properly when a time is input. If this file cannot be
% found, this function will try to create it by calling GETIGRFCOEFS.
% 
% The IGRF is a spherical harmonic expansion of the Earth's internal
% magnetic field. Currently, the IGRF model is valid between the years 1900
% and 2015. See the health warning for the IGRF model here:
% http://www.ngdc.noaa.gov/IAGA/vmod/igrfhw.html
% 
% Reference:
% International Association of Geomagnetism and Aeronomy, Working Group 
% V-MOD (2010), International Geomagnetic Reference Field: the eleventh
% generation, _Geophys. J. Int._, _183_(3), 1216-1230, 
% doi:10.1111/j.1365-246X.2010.04804.x.
% 
% Inputs:
%   -TIME: Time to get the magnetic field values either in MATLAB serial
%   date number format or a string that can be converted into MATLAB serial
%   date number format using DATENUM with no format specified (see
%   documentation of DATENUM for more information).
%   -COEFS: Instead of inputting a time, you can simply specify the proper
%   coefficients for the time you want by inputting in the first argument
%   the proper coefficient vector from igrfcoefs.mat.
%   -LATITUDE: Geocentric or geodetic latitude in degrees. **SCODIN**In radian
%   -LONGITUDE: Geocentric or geodetic longitude in degrees. **SCODIN**In radian
%   -ALTITUDE: For geodetic coordiates, the height in km above the Earth's
%   surface. For geocentric coordiates, the radius in km from the center of
%   the Earth.
%   -COORD: String specifying the coordinate system to use. Either
%   'geocentric' or 'geodetic' (optional, default is geodetic). Note that
%   only geodetic coordinates have been verified.
% 
% Outputs:
%   -BX: Northward component of the magnetic field in nanoteslas (nT).
%   -BY: Eastward component of the magnetic field in nT.
%   -BZ: Downward component of the magnetic field in nT.
%   -B: [BX(:), BY(:), BZ(:)].
% 
% See also: LOADIGRFCOEFS, GETIGRFCOEFS, IGRFLINE, DATENUM, IGRF11MAGM.

% Run IGRFS if all position inputs are scalars.
if isscalar(latitude) && isscalar(longitude) && isscalar(altitude)
        [Bn, Be, Bd] = igrfs(latitude, longitude, altitude);
end

if nargout <= 1
    Bn = [Bn(:), Be(:), Bd(:)];
end
%%%%%%%%%%%%%%%%%%%%%%%%%%%%%%%%%%%%%%%%%%%%%%%%%%%%%%%%%%%%%%%%%%%%%%%%%%%
%%%%%%%%%%%%%%%%%%%        IGRF scalar function.        %%%%%%%%%%%%%%%%%%%
%%%%%%%%%%%%%%%%%%%%%%%%%%%%%%%%%%%%%%%%%%%%%%%%%%%%%%%%%%%%%%%%%%%%%%%%%%%
function [Bn, Be, Bd] = igrfs(latitude, longitude, altitude)

% Fundamental constant.
Rearth_km = 6371.2;

%%% CHECK INPUT VALIDITY %%%
% Convert time to a datenumber if it is a string.
% if ischar(time)
%     time = datenum(time);
% end

% Check that the input coordinates are scalars.
if ~isscalar(latitude) || ~isscalar(longitude) || ~isscalar(altitude)
    error('igrf1:inputNotScalar', ...
        'The input coordinates must be scalars.');
end

%%% SPHERICAL COORDINATE CONVERSION %%%
% Convert the latitude, longitude, and altitude coordinates input into
% spherical coordinates r (radius), theta (inclination angle from +z axis),
% and phi (azimuth angle from +x axis).
% We want cos(theta) and sin(theta) rather than theta itself.
costheta = cos(((pi()/2) - latitude));
sintheta = sin(((pi()/2) - latitude));

% Convert from geodetic coordinates to geocentric coordinates if necessary.
% This method was adapted from igrf11syn, which was a conversion of the
% IGRF subroutine written in FORTRAN.

r = altitude;

% Convert longitude to radians.
phi = longitude; %Conversion in Simulink

%IGRF Coefficient

gh = [-29442	-1501	4797.1	-2445.1	3012.9	-2845.6	1676.7	-641.9	1350.7	-2352.3	-115.3	1225.6	244.9	582	-538.4	907.6	813.7	283.3	120.4	-188.7	-334.9	180.9	70.4	-329.5	-232.6	360.1	47.3	192.4	197	-140.9	-119.3	-157.5	16	4.1	100.2	70	67.7	-20.8	72.7	33.2	-129.9	58.9	-28.9	-66.7	13.2	7.3	-70.9	62.6	81.6	-76.1	-54.1	-6.8	-19.5	51.8	5.7	15	24.4	9.4	3.4	-2.8	-27.4	6.8	-2.2	24.2	8.8	10.1	-16.9	-18.3	-3.2	13.3	-20.6	-14.6	13.4	16.2	11.7	5.7	-15.9	-9.1	-2	2.1	5.4	8.8	-21.6	3.1	10.8	-3.3	11.8	0.7	-6.8	-13.3	-6.9	-0.1	7.8	8.7	1	-9.1	-4	-10.5	8.4	-1.9	-6.3	3.2	0.1	-0.4	0.5	4.6	-0.5	4.4	1.8	-7.9	-0.7	-0.6	2.1	-4.2	2.4	-2.8	-1.8	-1.2	-3.6	-8.7	3.1	-1.5	-0.1	-2.3	2	2	-0.7	-0.8	-1.1	0.6	0.8	-0.7	-0.2	0.2	-2.2	1.7	-1.4	-0.2	-2.5	0.4	-2	3.5	-2.4	-1.9	-0.2	-1.1	0.4	0.4	1.2	1.9	-0.8	-2.2	0.9	0.3	0.1	0.7	0.5	-0.1	-0.3	0.3	-0.4	0.2	0.2	-0.9	-0.9	-0.1	0	0.7	0	-0.9	-0.9	0.4	0.4	0.5	1.6	-0.5	-0.5	1	-1.2	-0.2	-0.1	0.8	0.4	-0.1	-0.1	0.3	0.4	0.1	0.5	0.5	-0.3	-0.4	-0.4	-0.3	-0.8];
gh = transpose(gh);
nmax = sqrt(numel(gh) + 1) - 1;
% We need cos(m*phi) and sin(m*phi) multiple times, so precalculate into a
% vector here:
cosphi = cos((1:nmax)*phi);
sinphi = sin((1:nmax)*phi);

Pmax = (nmax+1)*(nmax+2)/2;

%%% BEGIN MAGNETIC FIELD CALCULATION %%%
% Initialize variables used in for loop below.
Br = 0; Bt = 0; Bp = 0;
 P = zeros(1, Pmax);  P(1) = 1;  P(3) = sintheta;
dP = zeros(1, Pmax); dP(1) = 0; dP(3) = costheta;

% For this initial condition, the first if will result in n = 1, m = 0.
m = 1; n = 0; coefindex = 1;

a_r = (Rearth_km/r)^2;

% Increment through all the n's and m's. gh will be a vector with g
% followed by h for incrementing through n and m except when h would be
% redundant (i.e., when m = 0).
for Pindex = 2:Pmax
    
    % Increment to the next n when m becomes larger than n.
    if n < m
        m = 0;
        n = n + 1;
        a_r = a_r*(Rearth_km/r); % We need (Rearth_km./r)^(n+2)
    end
    
    % Calculate P and dP. They are given recursively according to:
    % 
    % P(0, 0) = 1, P(1, 1) = sin(theta) <- Specified above
    % P(n, n) = sqrt(1 - 1/(2n))*sin(theta)*P(n-1, n-1)
    % P(n, m) = (2n - 1)/sqrt(n^2 - m^2)*cos(theta)*P(n-1, m) -
    %     sqrt(((n-1)^2 - m^2) / (n^2 - m^2)) * P(n-2, m)
    % 
    % dP(0, 0) = 0, dP(1, 1) = cos(theta) <- Specified above
    % dP(n, n) = sqrt(1 - 1/(2n))*(sin(theta)*dP(n-1, n-1) +
    %     cos(theta)*P(n-1, n-1))
    % dP(n, m) = (2n - 1)/sqrt(n^2 - m^2)*(cos(theta)*dP(n-1, m) -
    %     sin(theta)*P(n-1, m)) - sqrt(((n-1)^2 - m^2)/(n^2 - m^2))*
    %     dP(n-2, m)
    if m < n && Pindex ~= 3 % (Pindex=3 is n=1, m=1, initial cond. above)
        last1n = Pindex - n;
        last2n = Pindex - 2*n + 1;
        P(Pindex) = (2*n - 1)/sqrt(n^2 - m^2)*costheta*P(last1n) - ...
            sqrt(((n-1)^2 - m^2) / (n^2 - m^2)) * P(last2n);
        dP(Pindex) = (2*n - 1)/sqrt(n^2 - m^2)*(costheta*dP(last1n) - ...
            sintheta*P(last1n)) - sqrt(((n-1)^2 - m^2) / (n^2 - m^2)) * ...
            dP(last2n);
    elseif Pindex ~= 3
        lastn = Pindex - n - 1;
        P(Pindex) = sqrt(1 - 1/(2*m))*sintheta*P(lastn);
        dP(Pindex) = sqrt(1 - 1/(2*m))*(sintheta*dP(lastn) + ...
            costheta*P(lastn));
    end
    
    % Calculate the magnetic field components as a running sum. Find
    % explicit expressions for these in Global Earth Physics: a Handbook of
    % Physical Constants by Thomas J. Aherns (1995), pg. 49. Link:
    % http://books.google.com/books?id=aqjU_NHyre4C&lpg=PP1&dq=Global%20
    % earth%20physics%3A%20a%20handbook%20of%20physical%20constants&pg=PA49
    % #v=onepage&q&f=false
    % (except equation 6 is missing a required 1/sin(theta) and m; correct
    % equations on page 5 (equations 3a-3c) of:
    % http://hanspeterschaub.info/Papers/UnderGradStudents/
    % MagneticField.pdf)
    if m == 0 % Implies h = 0, so only coefficient in gh is g
        coef = a_r*gh(coefindex); %*cos(0*phi) = 1
        Br = Br + (n+1)*coef*P(Pindex);
        Bt = Bt - coef*dP(Pindex);
        % Bp is 0 for m = 0.
        coefindex = coefindex + 1; % Only need to skip over g this time.
    else
        coef = a_r*(gh(coefindex)*cosphi(m) + gh(coefindex+1)*sinphi(m));
        Br = Br + (n+1)*coef*P(Pindex);
        Bt = Bt - coef*dP(Pindex);
        if sintheta == 0 % Use different formula when dividing by 0.
            Bp = Bp - costheta*a_r*(-gh(coefindex)*sinphi(m) + ...
                gh(coefindex+1)*cosphi(m))*dP(Pindex);
        else
            Bp = Bp - 1/sintheta*a_r*m*(-gh(coefindex)*sinphi(m) + ...
                gh(coefindex+1)*cosphi(m))*P(Pindex);
        end
        coefindex = coefindex + 2; % Skip over g and h this time.
    end
    
    % Increment m.
    m = m + 1;
    
end

% Convert from spherical to (x,y,z) = (North,East,Down).
Bn = -Bt;
Be = Bp;
Bd = -Br;

== matlab function TEST/Subsystem/MATLAB Function1 ==
  data: lat_d input; DCM_ined output; lon_i input
function DCM_ined = T_di(lat_d,lon_i)

clat = cos(lat_d);
slat = sin(lat_d);
clon = cos(lon_i);
slon = sin(lon_i);

DCM_ined = [-slat*clon -slat*slon clat;
            -slon clon 0;
            -clat*clon -clat*slon -slat];

== matlab function TEST/Disturbances1/ATMOSPHERIC DRAG/MATLAB Function ==
  data: h input; rho output
function rho = fcn(h)

%Reference altitude (km)

h_ref =linspace(250,500,7);

%Reference density (kg/m3)

rho_ref = [7.3e-11 4.1e-11 2.3e-11 1.38e-11,...
           8.33e-12 5.24e-12 3.29e-12];

%Interpolate based on altitude to find density   
       
rho = interp1(h_ref, rho_ref, h);
